simulink model "frist_order"  (R2023b)
settings: Solver=VariableStepAuto  StartTime=0.0  StopTime=10.0  RelTol=1e-3
settings Model: Creator=ascom  LastModifiedBy=ascom

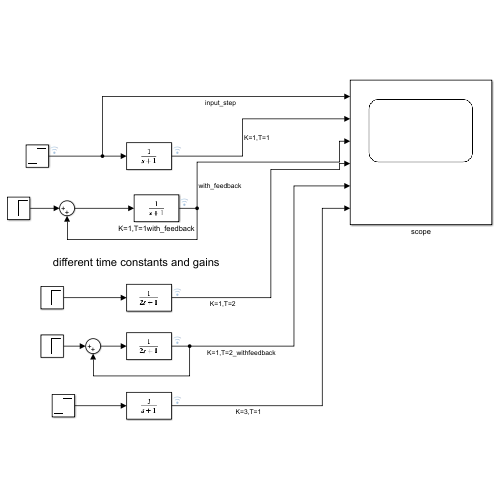
[thumbnail: Simulink's stored preview of the top-level diagram]
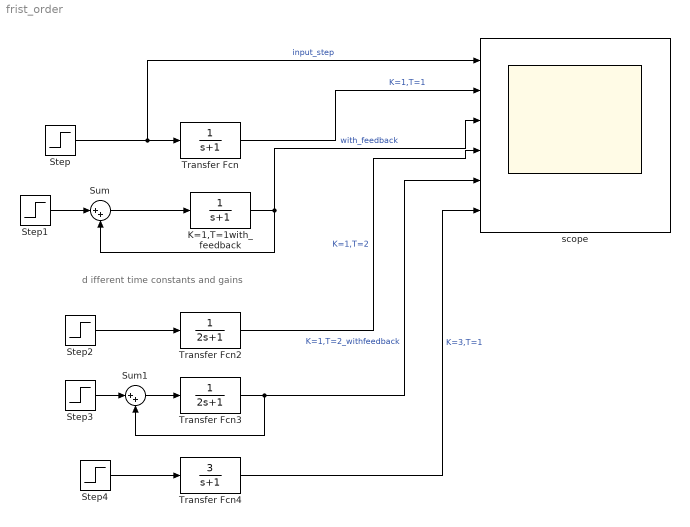
== system frist_order ==
  note: d ifferent time constants and gains
  K=1,T=1with_feedback : TransferFcn  Denominator=[1 1]
  Step{,1..4} (5 alike) : Step  SampleTime=0
  Sum : Sum  Inputs=|++
  Sum1 : Sum  Inputs=|++
  Transfer Fcn : TransferFcn  Denominator=[1 1]
  Transfer Fcn2 : TransferFcn  Denominator=[2 1]
  Transfer Fcn3 : TransferFcn  Denominator=[2 1]
  Transfer Fcn4 : TransferFcn  Numerator=[3]  Denominator=[1 1]
  scope : Scope  NumInputPorts=6
  wires:
  Step/1 -> scope/1, Transfer Fcn/1  "input_step"
  Sum/1 -> K=1,T=1with_feedback/1
  K=1,T=1with_feedback/1 -> Sum/2, scope/3  "with_feedback"
  Step1/1 -> Sum/1
  Step2/1 -> Transfer Fcn2/1
  Step4/1 -> Transfer Fcn4/1
  Transfer Fcn/1 -> scope/2  "K=1,T=1"
  Transfer Fcn2/1 -> scope/4  "K=1,T=2"
  Transfer Fcn3/1 -> scope/5, Sum1/2  "K=1,T=2_withfeedback"
  Transfer Fcn4/1 -> scope/6  "K=3,T=1"
  Step3/1 -> Sum1/1
  Sum1/1 -> Transfer Fcn3/1
